simulink model "GCS_Demo"  (R2021a)
settings: Solver=VariableStepAuto  StartTime=0.0  StopTime=inf  RelTol=1e-3
libraries: instrumentseriallib x2, etargetslib x1
settings Model: EnablePacing=on  Creator=Alireza  LastModifiedBy=Alireza

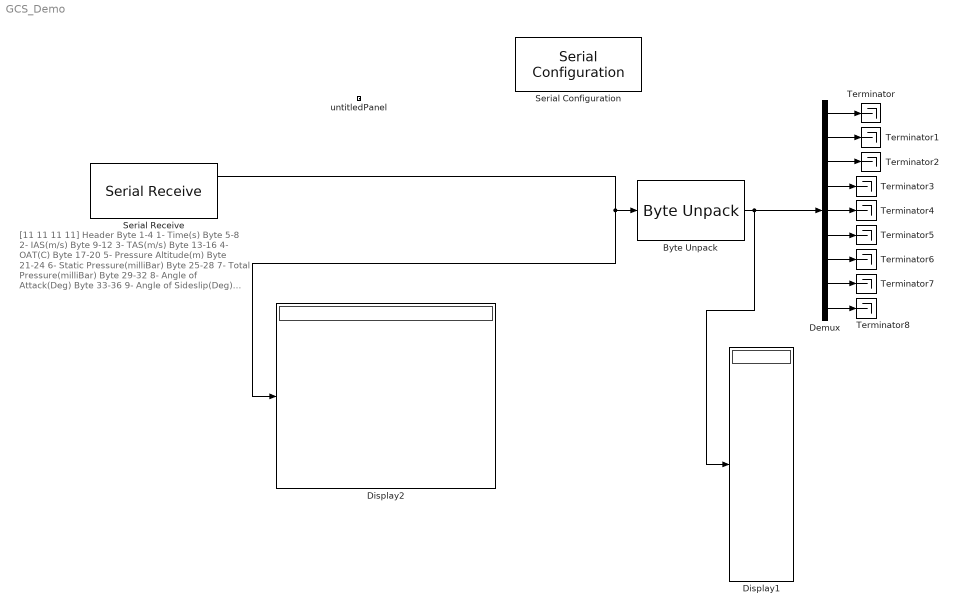
== system GCS_Demo ==
  note: [11 11 11 11] Header Byte 1-4
      | 1- Time(s) Byte 5-8
      | 2- IAS(m/s) Byte 9-12
      | 3- TAS(m/s) Byte 13-16
      | 4- OAT(C) Byte 17-20
      | 5- Pressure Altitude(m) Byte 21-24
      | 6- Static Pressure(milliBar) Byte 25-28
      | 7- Total Pressure(milliBar) Byte 29-32
      | 8- Angle of Attack(Deg) Byte 33-36
      | 9- Angle of Sideslip(Deg) Byte 37-40
      | [10 10 10 10] Terminator Byte 41-44
  Byte Unpack : etargetslib/Byte Unpack  dimensions={[9]}  datatypes={'single'}  byteAlign=1
  Demux : Demux  Outputs=9
  Display1 : Display
  Display2 : Display
  Serial Configuration : instrumentseriallib/Serial Configuration  Priority=-200000  Port=COM8  ComPort=COM8  BaudRate=57600  DataBits=8  Parity=none  StopBits=1  ByteOrder=little-endian  FlowControl=none  Timeout=10  SimulateUsing=Interpreted execution  BlockInModel=on
  Serial Receive : instrumentseriallib/Serial Receive  Priority=1  Port=COM8  ComPort=COM8  DataType=uint8  SaveDataType=uint8  ToggleHeader=on  Header=[11 11 11 11]  ToggleTerminator=on  Terminator=Custom terminator  CustomTerminator=[10 10 10 10]  ToggleDataSize=on  DataSize=[36]  EnableBlockingMode=off  ActionDataUnavailable=Output last received value  ActionWhenDataUnavailable=Output last received value  CustomValue=0  SampleTime=0.01  SimulateUsing=Interpreted execution  BlockInModel=on
  Terminator{,1..8} (9 alike) : Terminator
  untitledPanel : Subsystem  Tag=HiddenForWebPanel  IsWebBlockPanel=on
  wires:
  Serial Receive/1 -> Display2/1, Byte Unpack/1
  Byte Unpack/1 -> Display1/1, Demux/1
  Demux/1 -> Terminator/1
  Demux/2 -> Terminator1/1
  Demux/3 -> Terminator2/1
  Demux/4 -> Terminator3/1
  Demux/5 -> Terminator4/1
  Demux/6 -> Terminator5/1
  Demux/7 -> Terminator6/1
  Demux/8 -> Terminator7/1
  Demux/9 -> Terminator8/1

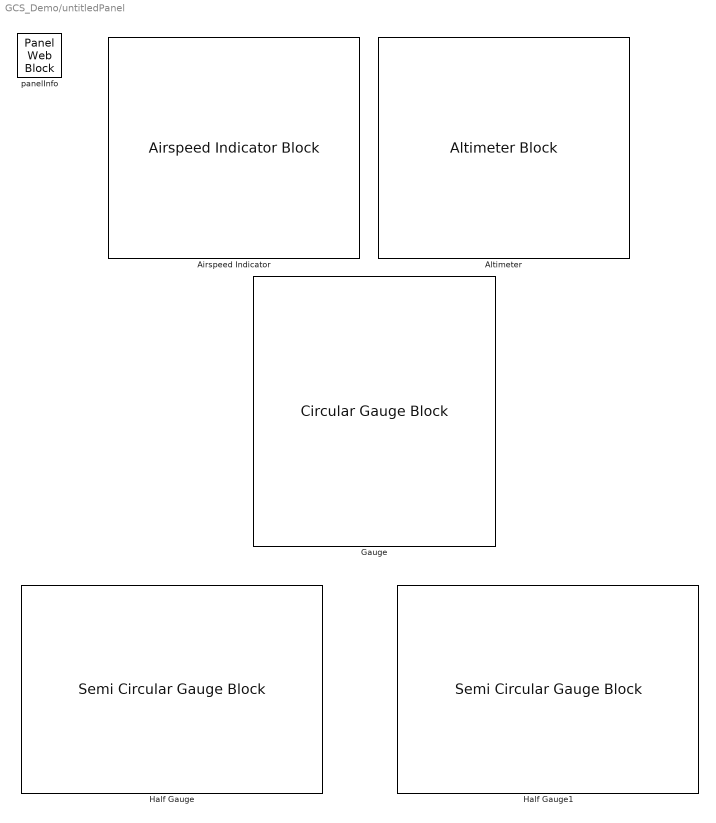
== system GCS_Demo/untitledPanel ==
  Airspeed Indicator : AirspeedIndicatorBlock  Tag=HiddenForWebPanel  PanelInfo="{\"panelId\":\"panelId-93f20305-647e-43b0-9893-948fd16e2aee\",\"type\":\"panelChild\",\"version\":\"2019b\",\"zIndex\":1500008}"
  Altimeter : AltimeterBlock  Tag=HiddenForWebPanel  PanelInfo="{\"panelId\":\"panelId-93f20305-647e-43b0-9893-948fd16e2aee\",\"type\":\"panelChild\",\"version\":\"2019b\",\"zIndex\":1500006}"
  Gauge : CircularGaugeBlock  Tag=HiddenForWebPanel  PanelInfo="{\"panelId\":\"panelId-93f20305-647e-43b0-9893-948fd16e2aee\",\"type\":\"panelChild\",\"version\":\"2019b\",\"zIndex\":1500004}"  ScaleMin=-20  ScaleMax=60
  Half Gauge : SemiCircularGaugeBlock  Tag=HiddenForWebPanel  PanelInfo="{\"panelId\":\"panelId-93f20305-647e-43b0-9893-948fd16e2aee\",\"type\":\"panelChild\",\"version\":\"2019b\",\"zIndex\":1500010}"  ScaleMin=-40  ScaleMax=+40
  Half Gauge1 : SemiCircularGaugeBlock  Tag=HiddenForWebPanel  PanelInfo="{\"panelId\":\"panelId-93f20305-647e-43b0-9893-948fd16e2aee\",\"type\":\"panelChild\",\"version\":\"2019b\",\"zIndex\":1500002}"  ScaleMin=-40  ScaleMax=+40
  panelInfo : PanelWebBlock  Tag=HiddenForWebPanel  PanelInfo="{\"compacted\":true,\"height\":1347,\"isActiveTab\":true,\"left\":1120,\"name\":\"Panel\",\"panelId\":\"panelId-93f20305-647e-43b0-9893-948fd16e2aee\",\"tabIndex\":0,\"tabbedSetId\":\"tabbedSet5987612390\",\"top\":343,\"type\":\"panel\",\"version\":\"2019b\",\"visible\":true,\"width\":1212,\"zIndex\":1500002}"  PanelSnapshot=<binary blob, 186184 chars, not shown>
